simulink model "poda"  (R2020a)
settings: Solver=ode45  StartTime=0.0  StopTime=500  RelTol=1e-3  EnableMultiTasking=on
values from neighbouring files (symbols this model uses):
  A1 = str2double(get(handles.edit5,'string'))    [Gui.m]
  A2 = str2double(get(handles.edit6,'string'))    [Gui.m]
  mi1 = str2double(get(handles.edit3,'string'))    [Gui.m]
  mi2 = str2double(get(handles.edit4,'string'))    [Gui.m]
  mu1 = str2double(get(handles.edit2,'string'))    [Gui.m]
settings Model: Creator=Sandra Knezevic  LastModifiedBy=Aldin
settings DataIOCC: LimitDataPoints=on  SaveFormat=Array  ReturnWorkspaceOutputs=off
settings OptimizationCC: LifeSpan=inf
settings DebuggingCC: SFUnexpectedBacktrackingDiag=warning  SFNoUnconditionalDefaultTransitionDiag=warning  SFExecutionAtInitializationDiag=none  ArithmeticOperatorsInVariantConditions=warning
settings HardwareCC: ProdBitPerPointer=32  ProdBitPerSizeT=32  ProdBitPerPtrDiffT=32  ProdLargestAtomicFloat=None  ProdIntDivRoundTo=Undefined  ProdEndianess=Unspecified  ProdWordSize=32  ProdHWDeviceType=32-bit Generic
settings ModelReferenceCC: PropagateSignalLabelsOutOfModel=off
settings SFSimCC: SimUseLocalCustomCode=off  CustomCodeUndefinedFunction=UseInterfaceOnly
settings RTWCC: RTWUseLocalCustomCode=off
settings CodeAppCC: StateflowObjectComments=on
settings GRTTargetCC: TargetLangStandard=C89/C90 (ANSI)
settings ConfigComp: CovMetricSettings=dw  CovHtmlReporting=on  CovSaveCumulativeToWorkspaceVar=on  CovSaveSingleToWorkspaceVar=on  CovExternalEMLEnable=off

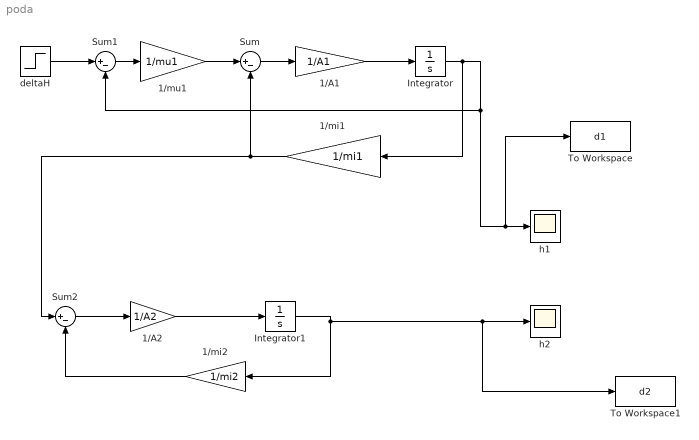
== system poda ==
  1/A1 : Gain  Gain=1/A1
  1/A2 : Gain  Gain=1/A2
  1/mi1 : Gain  Gain=1/mi1
  1/mi2 : Gain  Gain=1/mi2
  1/mu1 : Gain  Gain=1/mu1
  Integrator : Integrator  InitialCondition=1
  Integrator1 : Integrator  InitialCondition=1
  Sum : Sum  Inputs=|+-
  Sum1 : Sum  Inputs=|+-
  Sum2 : Sum  Inputs=|+-
  To Workspace : ToWorkspace  VariableName=d1  SampleTime=-1
  To Workspace1 : ToWorkspace  VariableName=d2  SampleTime=-1
  deltaH : Step  After=15  SampleTime=0
  h1 : Scope
  h2 : Scope
  wires:
  1/A1/1 -> Integrator/1
  1/mu1/1 -> Sum/1
  Sum/1 -> 1/A1/1
  Sum1/1 -> 1/mu1/1
  deltaH/1 -> Sum1/1
  Integrator/1 -> 1/mi1/1, To Workspace/1, h1/1, Sum1/2
  1/mi1/1 -> Sum/2, Sum2/1
  Sum2/1 -> 1/A2/1
  1/A2/1 -> Integrator1/1
  Integrator1/1 -> To Workspace1/1, h2/1, 1/mi2/1
  1/mi2/1 -> Sum2/2
